simulink model "sim5"  (R2023a)
settings: Solver=VariableStepAuto  StartTime=0  StopTime=10  FixedStep=0.01  RelTol=1e-8
undefined symbols (not defined in the file): A1, A2, A3, k, sw, T, w1, w2, w3
settings Model: Creator=vasil  LastModifiedBy=vasil

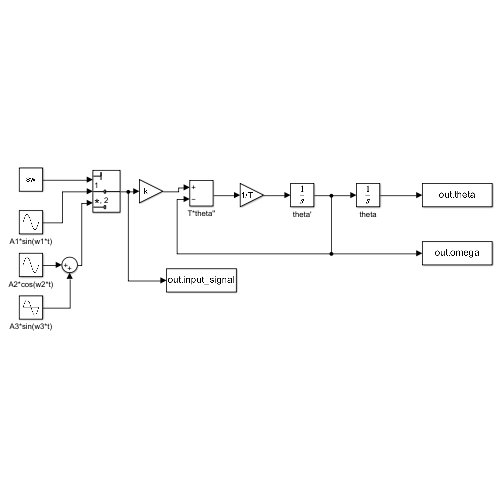
[thumbnail: Simulink's stored preview of the top-level diagram]
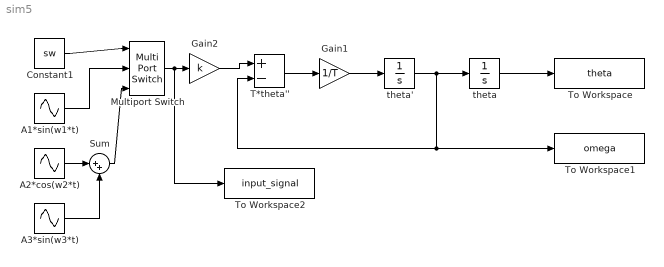
== system sim5 ==
  A1*sin(w1*t) : Sin  Amplitude=A1  Frequency=w1  SampleTime=0
  A2*cos(w2*t) : Sin  Amplitude=A2  Frequency=w2  Phase=pi/2  SampleTime=0
  A3*sin(w3*t) : Sin  Amplitude=A3  Frequency=w3  SampleTime=0
  Constant1 : Constant  Value=sw
  Gain1 : Gain  Gain=1/T
  Gain2 : Gain  Gain=k
  Multiport Switch : MultiPortSwitch  Inputs=2  SaturateOnIntegerOverflow=off  InputSameDT=off
  Sum : Sum  Inputs=|++
  T*theta'' : Sum  Inputs=+-
  To Workspace : ToWorkspace  VariableName=theta  SaveFormat=Timeseries  SampleTime=-1
  To Workspace1 : ToWorkspace  VariableName=omega  SaveFormat=Timeseries  SampleTime=-1
  To Workspace2 : ToWorkspace  VariableName=input_signal  SaveFormat=Timeseries  SampleTime=-1
  theta : Integrator
  theta' : Integrator
  wires:
  theta/1 -> To Workspace/1
  T*theta''/1 -> Gain1/1
  theta'/1 -> theta/1, To Workspace1/1, T*theta''/2
  Multiport Switch/1 -> To Workspace2/1, Gain2/1
  Constant1/1 -> Multiport Switch/1
  A1*sin(w1*t)/1 -> Multiport Switch/2
  A2*cos(w2*t)/1 -> Sum/1
  Sum/1 -> Multiport Switch/3
  A3*sin(w3*t)/1 -> Sum/2
  Gain1/1 -> theta'/1
  Gain2/1 -> T*theta''/1
